simulink model "VentilateurMODELE"  (R2022a)
settings: Solver=VariableStepAuto  StartTime=0.0  StopTime=12  RelTol=1e-3
undefined symbols (not defined in the file): a, b, c, d, f, p, r
settings Model: Creator=Ilyas ABDELLAOUI  LastModifiedBy=Ilyas ABDELLAOUI

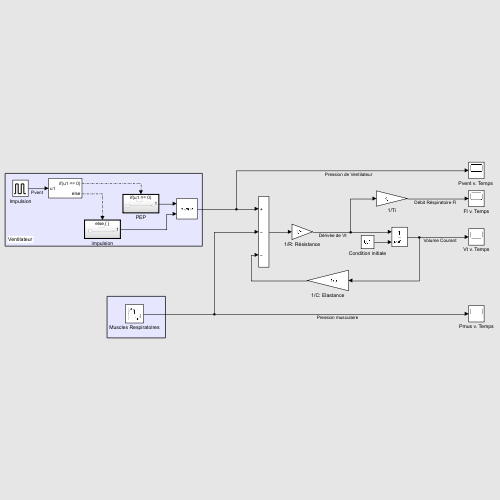
[thumbnail: Simulink's stored preview of the top-level diagram]
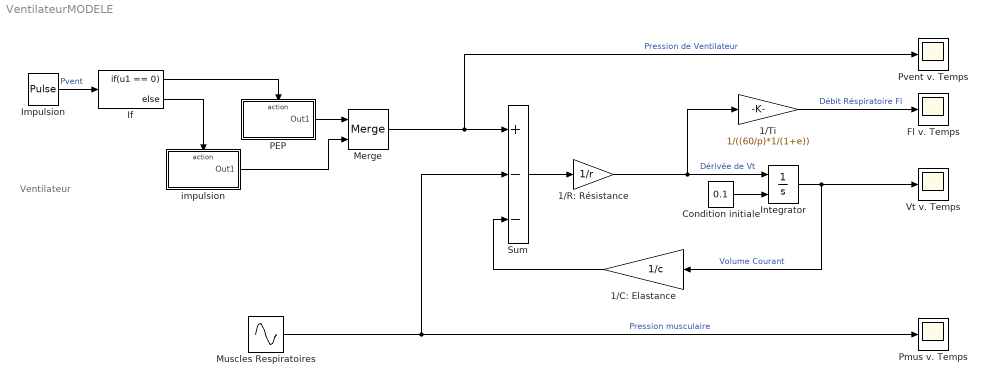
== system VentilateurMODELE ==
  note: Ventilateur
  1/C: Elastance : Gain  Gain=1/c
  1/R: Résistance : Gain  Gain=1/r
  1/Ti : Gain  Gain=1/((60/p)*1/(1+e))
  Condition initiale : Constant  Value=0.1
  Fl v. Temps : Scope
  If : If  IfExpression=u1 == 0
  Impulsion : DiscretePulseGenerator  PulseType=Time based  Amplitude=a  Period=60/p  PulseWidth=d
  Integrator : Integrator  InitialConditionSource=external
  Merge : Merge
  Muscles Respiratoires : Sin  Amplitude=f  SampleTime=0.01
  PEP : Subsystem  TreatAsAtomicUnit=on
  Pmus v. Temps : Scope
  "Pvent v. Temps " : Scope
  Sum : Sum  Inputs=+--
  Vt v. Temps : Scope
  impulsion : Subsystem  TreatAsAtomicUnit=on
  wires:
  Sum/1 -> 1/R: Résistance/1
  Integrator/1 -> Vt v. Temps/1, 1/C: Elastance/1  "Volume Courant"
  1/Ti/1 -> Fl v. Temps/1  "Débit Réspiratoire Fl"
  1/R: Résistance/1 -> Integrator/1, 1/Ti/1  "Dérivée de Vt"
  1/C: Elastance/1 -> Sum/3
  Condition initiale/1 -> Integrator/2
  Muscles Respiratoires/1 -> Sum/2, Pmus v. Temps/1  "Pression musculaire"
  impulsion/1(Out1) -> Merge/2
  If/2 -> impulsion/Action
  Impulsion/1 -> If/1  "Pvent"
  PEP/1(Out1) -> Merge/1
  If/1 -> PEP/Action
  Merge/1 -> "Pvent v. Temps "/1, Sum/1  "Pression de Ventilateur"

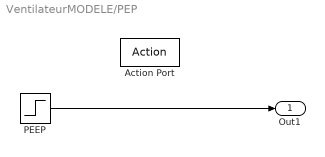
== system VentilateurMODELE/PEP ==
  Action Port : ActionPort  InitializeStates=reset  ActionPortLabel=if(u1 == 0)
  PEEP : Step  Time=0  After=b  SampleTime=0
  Out1 : Outport
  wires:
  PEEP/1 -> Out1/1

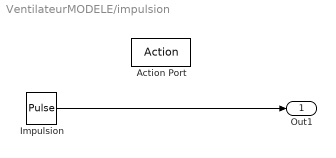
== system VentilateurMODELE/impulsion ==
  Action Port : ActionPort  InitializeStates=reset  ActionPortLabel=else
  Impulsion : DiscretePulseGenerator  PulseType=Time based  TimeSource=Use external signal  Amplitude=a  Period=60/p  PulseWidth=d
  Out1 : Outport
  wires:
  Impulsion/1 -> Out1/1
